simulink model "px4_controller_demo"  (R2022a)
settings: Solver=FixedStepAuto  StartTime=0.0  StopTime=inf  RelTol=1e-3  EnableMultiTasking=on
undefined symbols (not defined in the file): AUX, dev, DiscIntNeverNeededParam, dt, Main, pwm_output0, pwm_output1
libraries: simulink x8, px4lib x7, slpidlib x5, px4uORBlib x3, simulink_extras x2, sharedtransform x1, px4Sensorslib x1
settings Model: SimulationMode=external  ExtModeTrigDuration=10  Creator=The MathWorks, Inc.  LastModifiedBy=18395
settings SolverCC: AlgebraicLoopSolver=TrustRegion  PositivePriorityOrder=on  MaxZcPerStep=1
settings OptimizationCC: EnhancedBackFolding=on  PassReuseOutputArgsAs=Individual arguments  MaxStackSize=64  OptimizeBlockOrder=speed  DifferentSizesBufferReuse=on  OptimizationCustomize=off  EfficientTunableParamExpr=on
settings DebuggingCC: ParameterTunabilityLossMsg=error  UnconnectedInputMsg=warning  UnconnectedOutputMsg=warning  UnconnectedLineMsg=warning  SFMachineParentedDataDiag=warning  ArithmeticOperatorsInVariantConditions=warning
settings HardwareCC: ProdBitPerPointer=32  ProdBitPerSizeT=32  ProdBitPerPtrDiffT=32  ProdLargestAtomicInteger=Long  ProdLargestAtomicFloat=Double  ProdWordSize=32  ProdLongLongMode=on  ProdHWDeviceType=ARM Compatible->ARM Cortex
settings SFSimCC: MATLABDynamicMemAlloc=off  SimTargetLang=C++
settings RTWCC: SystemTargetFile=ert.tlc  HardwareBoard=PX4 Pixhawk 4  TLCOptions="-aInlineSetEventsForThisBaseRateFcn=TLC_FALSE -aSuppressMultiTaskScheduler=TLC_FALSE  -aRateBasedStepFcn=0"  TemplateMakefile=ert_default_tmf  GenerateReport=on  Toolchain=GNU Tools for PX4 Autopilots  IncludeHyperlinkInReport=on  LaunchReport=on  TargetLang=C++  GenerateTraceInfo=on  GenerateTraceReport=on  GenerateTraceReportSl=on  GenerateTraceReportSf=on  GenerateTraceReportEml=on  DLArmComputeVersion=19.05
settings CodeAppCC: ForceParamTrailComments=on  IgnoreCustomStorageClasses=off  OperatorAnnotations=on  SimulinkDataObjDesc=on  SFDataObjDesc=on  InsertBlockDesc=on
settings ERTTargetCC: ExtModeTransport=3  ExtModeStaticAlloc=on  ExtModeStaticAllocSize=1024  ExtModeMexFile=ext_xcp  ExtModeIntrfLevel=Level2 - Open

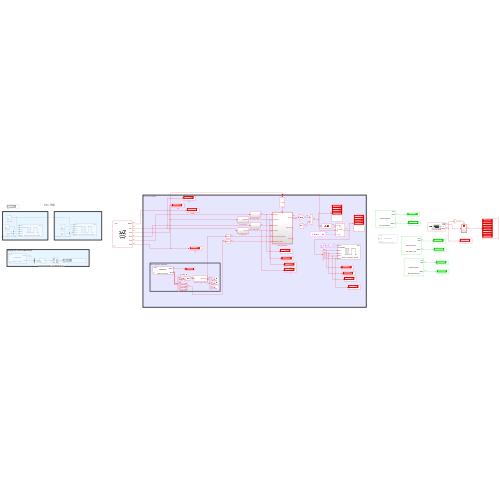
[thumbnail: Simulink's stored preview of the top-level diagram]
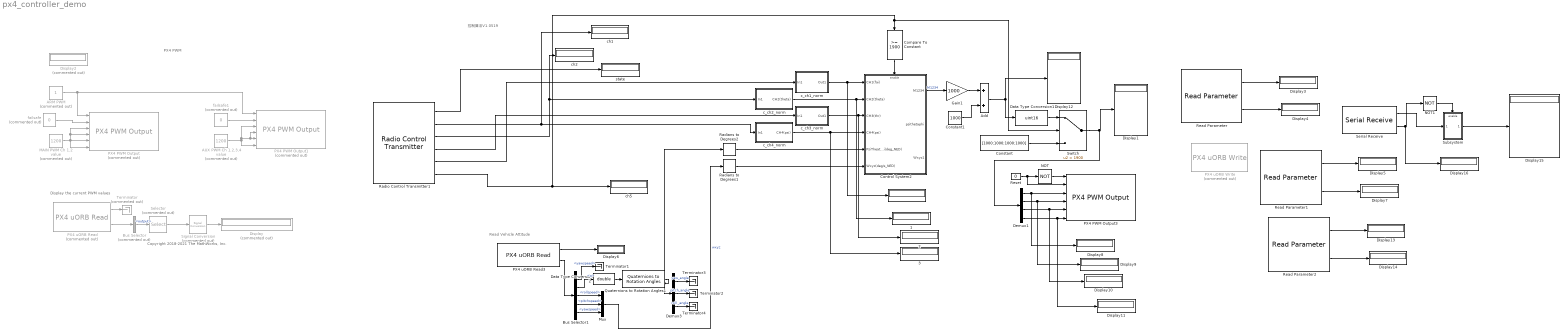
== system px4_controller_demo ==
  note: Copyright 2018-2021 The MathWorks, Inc.
  note: PX4 PWM
  note: Display the current PWM values
  note: 控制算法V1.0519
  note: Read Vehicle Attitude
    {,1..3} (4 alike) : Display
  ARM PWM : Constant  Commented=on  OutDataTypeStr=boolean  SampleTime=0.01
  AUX PWM Ch 1,2,3,4 value : Constant  Commented=on  Value=1200  OutDataTypeStr=uint16  SampleTime=0.01
  Add : Sum
  Bus Selector : BusSelector  Commented=on  OutputSignals=output
  Bus Selector1 : BusSelector  OutputSignals=yawspeed,q,rollspeed,pitchspeed,yawspeed
  Compare To Constant : simulink/Logic and Bit Operations/Compare To Constant  relop=>=  const=1900  OutDataTypeStr=boolean
  Constant : Constant  Value=[1000;1000;1000;1000]  OutDataTypeStr=uint16
  Constant1 : Constant  Value=1000  SampleTime=-1
  Control System2 : Subsystem
  Data Type Conversion1 : DataTypeConversion  OutDataTypeStr=uint16  SaturateOnIntegerOverflow=off  RndMeth=Floor
  Data Type Conversion2 : DataTypeConversion  OutDataTypeStr=double  SaturateOnIntegerOverflow=off  RndMeth=Floor
  Demux1 : Demux
  Demux3 : Demux  Outputs=3
  Display : Display  Commented=on
  Display{1,3..16} (15 alike) : Display
  Display2 : Display  Commented=on
  Gain1 : Gain  Gain=1000
  MAIN PWM Ch 1,2 value : Constant  Commented=on  Value=1200  OutDataTypeStr=uint16  SampleTime=0.01
  Mux : Mux  Inputs=3
  NOT : Logic  Operator=NOT  IconShape=distinctive  AllPortsSameDT=off  OutDataTypeStr=boolean
  NOT1 : Logic  Operator=NOT  IconShape=distinctive  AllPortsSameDT=off  OutDataTypeStr=boolean
  PX4 PWM Output : px4lib/PX4 PWM Output  Commented=on  pwmDevice=Main (/dev/pwm_output0)  pwmChannel1_=on  pwmChannel2_=on  pwmChannel3_=on  pwmChannel4_=on  pwmChannel5_=off  pwmChannel6_=off  pwmChannel7_=off  pwmChannel8_=off  forceTerminateFailsafe=off  outputErrorStatus=off
      settings: SourceProductBaseCode=PX4AUTOPILOTS
  PX4 PWM Output1 : px4lib/PX4 PWM Output  Commented=on  pwmDevice=AUX (/dev/pwm_output1)  pwmChannel1_=on  pwmChannel2_=on  pwmChannel3_=on  pwmChannel4_=on  pwmChannel5_=off  pwmChannel6_=off  pwmChannel7_=off  pwmChannel8_=off  forceTerminateFailsafe=off  outputErrorStatus=off
      settings: SourceProductBaseCode=PX4AUTOPILOTS
  PX4 PWM Output3 : px4lib/PX4 PWM Output  pwmDevice=Main (/dev/pwm_output0)  pwmChannel1_=on  pwmChannel2_=on  pwmChannel3_=on  pwmChannel4_=on  pwmChannel5_=off  pwmChannel6_=off  pwmChannel7_=off  pwmChannel8_=off  forceTerminateFailsafe=off  outputErrorStatus=off
      settings: SourceProductBaseCode=PX4AUTOPILOTS
  PX4 uORB Read : px4uORBlib/PX4 uORB Read  Commented=on  uORBTopic=actuator_outputs  selectInstance=actuator_outputs  SampleTime=0.01  BlockingMode=off  BlockTimeout=1e-3
      settings: SourceProductBaseCode=PX4AUTOPILOTS
  PX4 uORB Read3 : px4uORBlib/PX4 uORB Read  uORBTopic=vehicle_odometry  selectInstance=vehicle_odometry  SampleTime=0.01  BlockingMode=off  BlockTimeout=1e-3
      settings: SourceProductBaseCode=PX4AUTOPILOTS
  PX4 uORB Write : px4uORBlib/PX4 uORB Write  Commented=on  uORBTopic=vehicle_gps_position  selectInstance=vehicle_gps_position  MessageQueueLen=1
      settings: SourceProductBaseCode=PX4AUTOPILOTS
  Quaternions to Rotation Angles1 : sharedtransform/Quaternions to Rotation Angles  rotationOrder=ZYX  aMode=aMode
      settings: SourceProductBaseCode=AE,PW,DR,MT,VE
  Radians to Degrees1 : simulink_extras/Transformations/Radians to Degrees
  Radians to Degrees2 : simulink_extras/Transformations/Radians to Degrees
  Radio Control Transmitter1 : px4Sensorslib/Radio Control Transmitter  channel1=on  channel2=on  channel3=on  channel4=on  channel5=on  channel6=off  channel7=off  channel8=off  channel_count=off  rssi=off  rc_input_source=off  timestamp_last_signal=off  time_stamp=off  sampleTime=-1  BlockingMode=off  BlockTimeout=5
      settings: SourceProductBaseCode=PX4AUTOPILOTS
  Read Parameter : px4lib/Read Parameter  ParameterName=MC_ROLLRATE_I  DataType=FLOAT  SampleTime=0.5
      settings: SourceProductBaseCode=PX4AUTOPILOTS
  Read Parameter1 : px4lib/Read Parameter  ParameterName=FW_MAN_P_SC  DataType=FLOAT  SampleTime=0.5
      settings: SourceProductBaseCode=PX4AUTOPILOTS
  Read Parameter2 : px4lib/Read Parameter  ParameterName=MC_ROLLRATE_K  DataType=FLOAT  SampleTime=0.5
      settings: SourceProductBaseCode=PX4AUTOPILOTS
  Reset : Constant  Value=0  OutDataTypeStr=boolean
  Selector : Selector  Commented=on  InputPortWidth=16  IndexOptions=Index vector (dialog)  Indices=[1 2]  OutputSizes=1
  Serial Receive : px4lib/Serial Receive  SCIModule=/dev/ttyS2  DataType=double  DataLength=8  OutputStatus=on  SampleTime=-1  BlockingMode=off  PartialData=off  Timeout=5
      settings: SourceProductBaseCode=PX4AUTOPILOTS
  Signal Conversion : SignalConversion  Commented=on  OverrideOpt=off
  Subsystem : Subsystem
  Switch : Switch  Criteria=u2 > Threshold  Threshold=1900  SaturateOnIntegerOverflow=off  InputSameDT=off
  Terminator : Terminator  Commented=on
  Terminator{1..4} (4 alike) : Terminator
  c_ch1_norm : Subsystem
  c_ch2_norm : Subsystem
  c_ch3_norm : Subsystem
  c_ch4_norm : Subsystem
  ch1 : Display
  ch2 : Display
  ch5 : Display
  failsafe : Constant  Commented=on  Value=0  OutDataTypeStr=boolean  SampleTime=0.01
  failsafe1 : Constant  Commented=on  Value=0  OutDataTypeStr=boolean  SampleTime=0.01
  state : Display
  wires:
  failsafe/1 -> PX4 PWM Output/2
  MAIN PWM Ch 1,2 value/1 -> PX4 PWM Output/6, PX4 PWM Output/4, PX4 PWM Output/3, PX4 PWM Output/5
  PX4 uORB Read/1 -> Terminator/1
  PX4 uORB Read/2 -> Bus Selector/1
  Bus Selector/1 -> Selector/1  "<output>"
  Selector/1 -> Signal Conversion/1
  failsafe1/1 -> PX4 PWM Output1/2
  ARM PWM/1 -> PX4 PWM Output1/1, PX4 PWM Output/1
  AUX PWM Ch 1,2,3,4 value/1 -> PX4 PWM Output1/3, PX4 PWM Output1/5, PX4 PWM Output1/4, PX4 PWM Output1/6
  Signal Conversion/1 -> Display/1
  Bus Selector1/4 -> Mux/2  "<pitchspeed>"
  Radio Control Transmitter1/5 -> c_ch1_norm/1(In1)
  Gain1/1 -> Add/1
  Radio Control Transmitter1/4 -> c_ch3_norm/1(In1)
  Reset/1 -> PX4 PWM Output3/2, NOT/1
  Radio Control Transmitter1/1 -> state/1
  Demux3/2 -> Terminator2/1  "pitch_angle"
  PX4 uORB Read3/2 -> Bus Selector1/1
  Demux1/3 -> Display10/1, PX4 PWM Output3/5
  Demux1/4 -> Display11/1, PX4 PWM Output3/6
  NOT/1 -> PX4 PWM Output3/1
  Quaternions to Rotation Angles1/1 -> Demux3/1, Radians to Degrees2/1
  Data Type Conversion2/1 -> Quaternions to Rotation Angles1/1
  Demux1/1 -> Display8/1, PX4 PWM Output3/3
  Demux3/3 -> Terminator4/1  "roll _angle"
  Control System2/1(M1234) -> Gain1/1  "M1234"
  Radio Control Transmitter1/2 -> c_ch4_norm/1(In1), ch1/1
  Radians to Degrees2/1 -> Control System2/5(PsiTheatphi(deg_NED))
  Mux/1 -> Radians to Degrees1/1  "wxyz"
  PX4 uORB Read3/1 -> Display6/1
  Radians to Degrees1/1 -> Control System2/6(Wxyz(deg/s_NED))
  Data Type Conversion1/1 -> Switch/1
  Bus Selector1/3 -> Mux/1  "<rollspeed>"
  Add/1 -> Data Type Conversion1/1, Display12/1
  Bus Selector1/2 -> Data Type Conversion2/1  "<q>"
  Constant1/1 -> Add/2
  Demux3/1 -> Terminator3/1  "yaw_angle"
  Radio Control Transmitter1/3 -> c_ch2_norm/1(In1), ch2/1
  Bus Selector1/5 -> Mux/3  "<yawspeed>"
  Bus Selector1/1 -> Terminator1/1  "<yawspeed>"
  c_ch3_norm/1(Out1) -> "  2"/1, Control System2/3(CH3(thr))
  c_ch2_norm/1(CH2(theta)) -> "  1"/1, Control System2/2(CH2(theta))
  c_ch4_norm/1(CH4(psi)) -> "  3"/1, Control System2/4(CH4(psi))
  c_ch1_norm/1(Out1) -> "  "/1, Control System2/1(CH1(fai))
  Demux1/2 -> Display9/1, PX4 PWM Output3/4
  Radio Control Transmitter1/6 -> ch5/1, Compare To Constant/1, Switch/2
  Compare To Constant/1 -> Control System2/Enable
  Switch/1 -> Demux1/1, Display1/1
  Constant/1 -> Switch/3
  Read Parameter/1 -> Display3/1
  Read Parameter/2 -> Display4/1
  Read Parameter1/2 -> Display7/1
  Read Parameter1/1 -> Display5/1
  Read Parameter2/1 -> Display13/1
  Read Parameter2/2 -> Display14/1
  Serial Receive/2 -> Display16/1, NOT1/1
  Serial Receive/1 -> Subsystem/1(In1)
  Subsystem/1(Out1) -> Display15/1
  NOT1/1 -> Subsystem/Enable

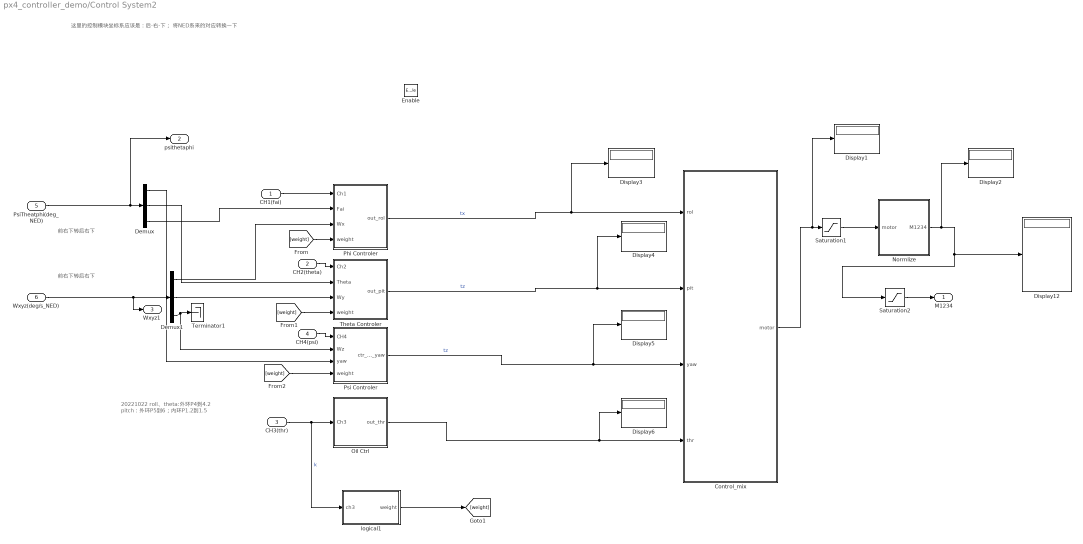
== system px4_controller_demo/Control System2 ==
  note: 20221022
      | roll、theta:外环P4到4.2
      | pitch：外环P5到6；内环P1.2到1.5
  note: 前右下转后右下
  note: 这里的控制模块坐标系应该是：后-右-下；
      | 将NED系来的对应转换一下
  note: 前右下转后右下
  CH1(fai) : Inport
  CH2(theta) : Inport  Port=2
  CH3(thr) : Inport  Port=3
  CH4(psi) : Inport  Port=4
  PsiTheatphi(deg_NED) : Inport  Port=5
  Wxyz(deg/s_NED) : Inport  Port=6
  Enable : EnablePort
  Control_mix : MATLAB Function  TreatAsAtomicUnit=on
  Demux : Demux  Outputs=3
  Demux1 : Demux  Outputs=3
  Display{1..6,12} (7 alike) : Display
  Normlize : Subsystem
  Oil Ctrl : Subsystem
  Phi Controler : Subsystem
  Psi Controler : Subsystem
  Saturation1 : Saturate  UpperLimit=1000  LowerLimit=0
  Saturation2 : Saturate  UpperLimit=1  LowerLimit=0
  Terminator1 : Terminator
  Theta Controler : Subsystem
  logical1 : Subsystem
  M1234 : Outport
  psithetaphi : Outport  Port=2
  Wxyz1 : Outport  Port=3
  wires:
  Demux1/3 -> Psi Controler/2(Wz), Terminator1/1
  Wxyz(deg/s_NED)/1 -> Wxyz1/1, Demux1/1
  PsiTheatphi(deg_NED)/1 -> psithetaphi/1, Demux/1
  CH2(theta)/1 -> Theta Controler/1(Ch2)
  CH4(psi)/1 -> Psi Controler/1(CH4)
  CH1(fai)/1 -> Phi Controler/1(Ch1)
  Demux1/1 -> Phi Controler/3(Wx)
  Demux1/2 -> Theta Controler/3(Wy)
  Demux/3 -> Phi Controler/2(Fai)
  Demux/2 -> Theta Controler/2(Theta)
  Saturation1/1 -> Normlize/1(motor)
  Normlize/1(M1234) -> Display2/1, Display12/1, Saturation2/1
  Saturation2/1 -> M1234/1
  Control_mix/1(motor) -> Display1/1, Saturation1/1
  Psi Controler/1(ctr_out_yaw) -> Display5/1, Control_mix/3(yaw)  "tz"
  Phi Controler/1(out_rol) -> Display3/1, Control_mix/1(rol)  "tx"
  Theta Controler/1(out_pit) -> Display4/1, Control_mix/2(pit)  "tz"
  Demux/1 -> Psi Controler/3(yaw)
  CH3(thr)/1 -> logical1/1(ch3), Oil Ctrl/1(Ch3)  "k"
  logical1/1(weight) -> [weight]
  [weight] -> Phi Controler/4(weight)
  [weight] -> Theta Controler/4(weight)
  [weight] -> Psi Controler/4(weight)
  Oil Ctrl/1(out_thr) -> Display6/1, Control_mix/4(thr)

== system px4_controller_demo/Subsystem ==
  In1 : Inport
  Enable : EnablePort
  Out1 : Outport
  wires:
  In1/1 -> Out1/1

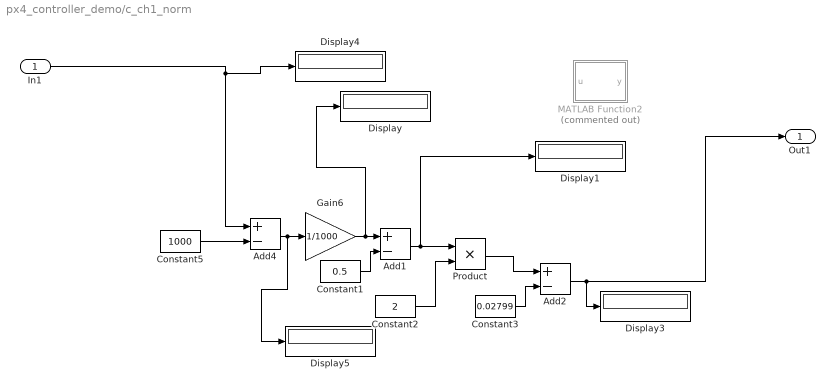
== system px4_controller_demo/c_ch1_norm ==
  In1 : Inport
  Add1 : Sum  Inputs=+-
  Add2 : Sum  Inputs=+-
  Add4 : Sum  Inputs=+-  AccumDataTypeStr=uint16
  Constant1 : Constant  Value=0.5
  Constant2 : Constant  Value=2  OutDataTypeStr=uint16
  Constant3 : Constant  Value=0.02799  OutDataTypeStr=uint16
  Constant5 : Constant  Value=1000  OutDataTypeStr=uint16
  Display{,1,3..5} (5 alike) : Display
  Gain6 : Gain  Gain=1/1000
  MATLAB Function2 : MATLAB Function  Commented=on  TreatAsAtomicUnit=on
  Product : Product
  Out1 : Outport
  wires:
  Add4/1 -> Display5/1, Gain6/1
  Constant5/1 -> Add4/2
  Gain6/1 -> Display/1, Add1/1
  In1/1 -> Display4/1, Add4/1
  Constant1/1 -> Add1/2
  Add1/1 -> Display1/1, Product/1
  Constant2/1 -> Product/2
  Product/1 -> Add2/1
  Constant3/1 -> Add2/2
  Add2/1 -> Display3/1, Out1/1

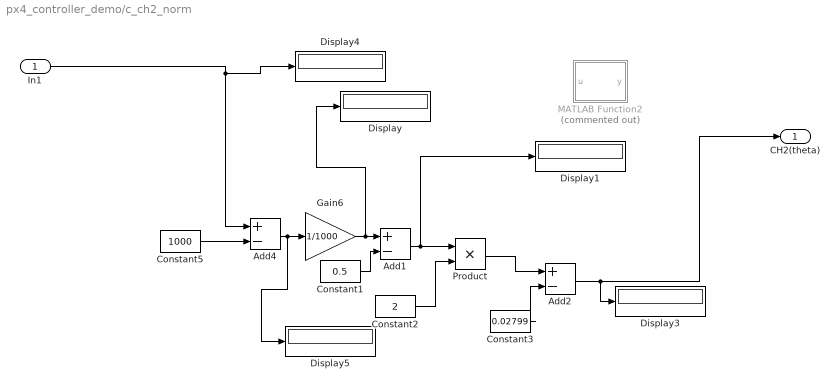
== system px4_controller_demo/c_ch2_norm ==
  In1 : Inport
  Add1 : Sum  Inputs=+-
  Add2 : Sum  Inputs=+-
  Add4 : Sum  Inputs=+-  AccumDataTypeStr=uint16
  Constant1 : Constant  Value=0.5
  Constant2 : Constant  Value=2  OutDataTypeStr=uint16
  Constant3 : Constant  Value=0.02799  OutDataTypeStr=uint16
  Constant5 : Constant  Value=1000  OutDataTypeStr=uint16
  Display{,1,3..5} (5 alike) : Display
  Gain6 : Gain  Gain=1/1000
  MATLAB Function2 : MATLAB Function  Commented=on  TreatAsAtomicUnit=on
  Product : Product
  CH2(theta) : Outport
  wires:
  Constant1/1 -> Add1/2
  Add1/1 -> Display1/1, Product/1
  Gain6/1 -> Display/1, Add1/1
  In1/1 -> Display4/1, Add4/1
  Add4/1 -> Display5/1, Gain6/1
  Constant2/1 -> Product/2
  Constant5/1 -> Add4/2
  Constant3/1 -> Add2/2
  Product/1 -> Add2/1
  Add2/1 -> Display3/1, CH2(theta)/1

== system px4_controller_demo/c_ch3_norm ==
  In1 : Inport
  Add2 : Sum  Inputs=+-
  Add4 : Sum  Inputs=+-  AccumDataTypeStr=uint16
  Constant3 : Constant  Value=0.095  OutDataTypeStr=uint16
  Constant5 : Constant  Value=1000  OutDataTypeStr=uint16
  Display : Display
  Display4 : Display
  Gain6 : Gain  Gain=1/1000
  Out1 : Outport
  wires:
  In1/1 -> Display4/1, Add4/1
  Add4/1 -> Gain6/1
  Constant5/1 -> Add4/2
  Constant3/1 -> Add2/2
  Gain6/1 -> Add2/1
  Add2/1 -> Display/1, Out1/1

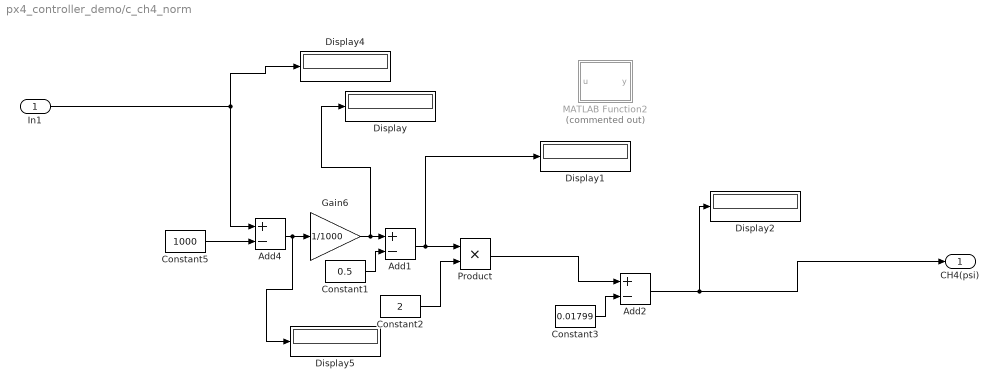
== system px4_controller_demo/c_ch4_norm ==
  In1 : Inport
  Add1 : Sum  Inputs=+-
  Add2 : Sum  Inputs=+-
  Add4 : Sum  Inputs=+-  AccumDataTypeStr=uint16
  Constant1 : Constant  Value=0.5
  Constant2 : Constant  Value=2  OutDataTypeStr=uint16
  Constant3 : Constant  Value=0.01799  OutDataTypeStr=uint16
  Constant5 : Constant  Value=1000  OutDataTypeStr=uint16
  Display{,1..2,4..5} (5 alike) : Display
  Gain6 : Gain  Gain=1/1000
  MATLAB Function2 : MATLAB Function  Commented=on  TreatAsAtomicUnit=on
  Product : Product
  CH4(psi) : Outport
  wires:
  Constant1/1 -> Add1/2
  Add1/1 -> Display1/1, Product/1
  Gain6/1 -> Display/1, Add1/1
  In1/1 -> Display4/1, Add4/1
  Add4/1 -> Display5/1, Gain6/1
  Constant2/1 -> Product/2
  Constant5/1 -> Add4/2
  Constant3/1 -> Add2/2
  Product/1 -> Add2/1
  Add2/1 -> Display2/1, CH4(psi)/1

== system px4_controller_demo/Control System2/Normlize ==
  motor : Inport
  Constant : Constant  Value=1000
  Divide : Product  Inputs=*/
  M1234 : Outport
  wires:
  Constant/1 -> Divide/2
  motor/1 -> Divide/1
  Divide/1 -> M1234/1

== system px4_controller_demo/Control System2/Oil Ctrl ==
  note: ch3油门归一化为[0 1,若ch3开度高于0.4，油门量足够俯仰滚转才能驱的动]
  Ch3 : Inport
  Gain : Gain  Gain=1000
  Max ExpRate1 : Saturate  UpperLimit=1000  LowerLimit=0
  out_thr : Outport
  wires:
  Ch3/1 -> Gain/1  "k"
  Max ExpRate1/1 -> out_thr/1
  Gain/1 -> Max ExpRate1/1

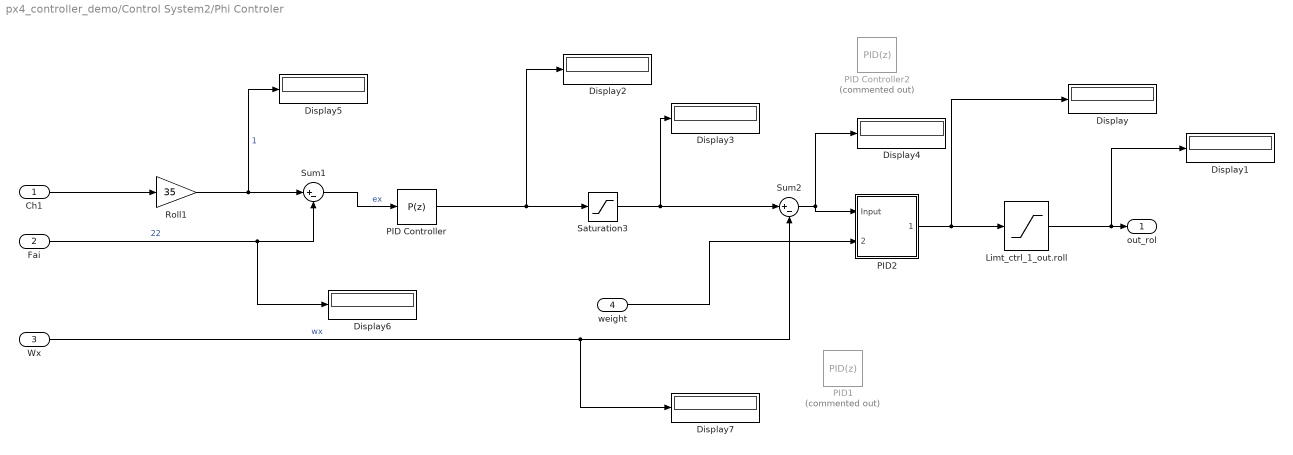
== system px4_controller_demo/Control System2/Phi Controler ==
  Ch1 : Inport
  Fai : Inport  Port=2
  Wx : Inport  Port=3
  weight : Inport  Port=4
  Display{,1..7} (8 alike) : Display
  Limt_ctrl_1_out.roll : Saturate  UpperLimit=1000  LowerLimit=-1000
  PID Controller : slpidlib/PID Controller  Controller=P  Form=Parallel  TimeDomain=Discrete-time  UseExternalTs=off  SampleTime=-1  IntegratorMethod=Forward Euler  FilterMethod=Forward Euler  ControllerParametersSource=internal  P=4  I=1  UseKiTs=off  D=0  N=100  UseFilter=on  TunerSelectOption=Transfer Function Based (PID Tuner App)  InitialConditionSource=internal  InitialConditionForIntegrator=0  InitialConditionForFilter=0  DifferentiatorICPrevScaledInput=0  ExternalReset=none  TrackingMode=off  Kt=1  LimitOutput=off  SatLimitsSource=internal  UpperSaturationLimit=inf  LowerSaturationLimit=-inf  LinearizeAsGain=on  AntiWindupMode=none  Kb=1  POutMin=[]  POutMax=[]  IOutMin=[]  IOutMax=[]  DOutMin=[]  DOutMax=[]  NOutMin=[]  NOutMax=[]  SumOutMin=[]  SumOutMax=[]  SaturationOutMin=[]  SaturationOutMax=[]  PParamMin=[]  PParamMax=[]  IParamMin=[]  IParamMax=[]  DParamMin=[]  DParamMax=[]  NParamMin=[]  NParamMax=[]  KbParamMin=[]  KbParamMax=[]  KtParamMin=[]  KtParamMax=[]  KbOutMin=[]  KbOutMax=[]  KtOutMin=[]  KtOutMax=[]  IntegratorOutMin=[]  IntegratorOutMax=[]  FilterOutMin=[]  FilterOutMax=[]  SumI1OutMin=[]  SumI1OutMax=[]  SumI2OutMin=[]  SumI2OutMax=[]  SumI3OutMin=[]  SumI3OutMax=[]  SumI4OutMin=[]  SumI4OutMax=[]  SumDOutMin=[]  SumDOutMax=[]  DifferentiatorOutMin=[]  DifferentiatorOutMax=[]  FilterDiffOutCoefMin=[]  FilterDiffOutCoefMax=[]  ReciprocalOutMin=[]  ReciprocalOutMax=[]  SumDenOutMin=[]  SumDenOutMax=[]  SumNumOutMin=[]  SumNumOutMax=[]  DivideOutMin=[]  DivideOutMax=[]  UdiffTsProdOutMin=[]  UdiffTsProdOutMax=[]  NTsProdOutMin=[]  NTsProdOutMax=[]  UintegralTsProdOutMin=[]  UintegralTsProdOutMax=[]  UngainTsProdOutMin=[]  UngainTsProdOutMax=[]  IntegratorContinuousStateAttributes=''  IntegratorStateMustResolveToSignalObject=off  IntegratorRTWStateStorageClass=Auto  FilterContinuousStateAttributes=''  FilterStateMustResolveToSignalObject=off  FilterRTWStateStorageClass=Auto  ParallelPVariant=InternalParameters  IdealPVariant=Disabled  IVariant=Disabled  DVariant=Disabled  IntegratorVariant=Disabled  SatVariant=Disabled  AWVariant=Disabled  PCopyVariant=Disabled  TRVariant=Disabled  FdbkBlocksVariant=Forward  IdealPFdbkVariant=Disabled  SatFdbkVariant=Disabled  DerivativeFilterVariant=Disabled  NVariant=Disabled  NCopyVariant=Disabled_SignalSpec  FilterICVariant=Disabled  IntegratorICVariant=Disabled  ExternalResetVariant=Disabled  TRSumVariant=Passthrough  SumFdbkVariant=Disabled  SumVariant=Passthrough_P  TsampFilterVariant=InternalTs  TsampNgainVariant=Passthrough  TsampIntegralVariant=Disabled_SignalSpec  ExternalSaturationOutDataTypeStr=Inherit: Same as second input  aMode=0
  PID Controller2 : slpidlib/PID Controller  Commented=on  Controller=PID  Form=Parallel  TimeDomain=Discrete-time  UseExternalTs=off  SampleTime=-1  IntegratorMethod=Forward Euler  FilterMethod=Forward Euler  ControllerParametersSource=internal  P=0.8  I=1.2  UseKiTs=off  D=0.03  N=100  UseFilter=on  TunerSelectOption=Transfer Function Based (PID Tuner App)  InitialConditionSource=internal  InitialConditionForIntegrator=0  InitialConditionForFilter=0  DifferentiatorICPrevScaledInput=0  ExternalReset=none  TrackingMode=off  Kt=1  LimitOutput=off  SatLimitsSource=internal  UpperSaturationLimit=inf  LowerSaturationLimit=-inf  LinearizeAsGain=on  AntiWindupMode=none  Kb=1  POutMin=[]  POutMax=[]  IOutMin=[]  IOutMax=[]  DOutMin=[]  DOutMax=[]  NOutMin=[]  NOutMax=[]  SumOutMin=[]  SumOutMax=[]  SaturationOutMin=[]  SaturationOutMax=[]  PParamMin=[]  PParamMax=[]  IParamMin=[]  IParamMax=[]  DParamMin=[]  DParamMax=[]  NParamMin=[]  NParamMax=[]  KbParamMin=[]  KbParamMax=[]  KtParamMin=[]  KtParamMax=[]  KbOutMin=[]  KbOutMax=[]  KtOutMin=[]  KtOutMax=[]  IntegratorOutMin=[]  IntegratorOutMax=[]  FilterOutMin=[]  FilterOutMax=[]  SumI1OutMin=[]  SumI1OutMax=[]  SumI2OutMin=[]  SumI2OutMax=[]  SumI3OutMin=[]  SumI3OutMax=[]  SumI4OutMin=[]  SumI4OutMax=[]  SumDOutMin=[]  SumDOutMax=[]  DifferentiatorOutMin=[]  DifferentiatorOutMax=[]  FilterDiffOutCoefMin=[]  FilterDiffOutCoefMax=[]  ReciprocalOutMin=[]  ReciprocalOutMax=[]  SumDenOutMin=[]  SumDenOutMax=[]  SumNumOutMin=[]  SumNumOutMax=[]  DivideOutMin=[]  DivideOutMax=[]  UdiffTsProdOutMin=[]  UdiffTsProdOutMax=[]  NTsProdOutMin=[]  NTsProdOutMax=[]  UintegralTsProdOutMin=[]  UintegralTsProdOutMax=[]  UngainTsProdOutMin=[]  UngainTsProdOutMax=[]  IntegratorContinuousStateAttributes=''  IntegratorStateMustResolveToSignalObject=off  IntegratorRTWStateStorageClass=Auto  FilterContinuousStateAttributes=''  FilterStateMustResolveToSignalObject=off  FilterRTWStateStorageClass=Auto  ParallelPVariant=InternalParameters  IdealPVariant=Disabled  IVariant=InternalParameters  DVariant=InternalParameters  IntegratorVariant=Discrete  SatVariant=Disabled  AWVariant=Passthrough  PCopyVariant=Disabled  TRVariant=Disabled  FdbkBlocksVariant=Forward  IdealPFdbkVariant=Disabled  SatFdbkVariant=Disabled  DerivativeFilterVariant=ForwardEulerFilter  NVariant=InternalParameters  NCopyVariant=Disabled  FilterICVariant=InternalICsFilter  IntegratorICVariant=InternalICs  ExternalResetVariant=Disabled  TRSumVariant=Passthrough  SumFdbkVariant=Disabled  SumVariant=Sum_PID  TsampFilterVariant=InternalTs  TsampNgainVariant=Passthrough  TsampIntegralVariant=Passthrough  ExternalSaturationOutDataTypeStr=Inherit: Same as second input  aMode=0
  PID1 : slpidlib/PID Controller  Commented=on  Controller=PID  Form=Parallel  TimeDomain=Discrete-time  UseExternalTs=off  SampleTime=-1  IntegratorMethod=Backward Euler  FilterMethod=Forward Euler  ControllerParametersSource=internal  P=0.8  I=1.2  UseKiTs=off  D=0.03  N=50  UseFilter=on  TunerSelectOption=Transfer Function Based (PID Tuner App)  InitialConditionSource=internal  InitialConditionForIntegrator=0  InitialConditionForFilter=0  DifferentiatorICPrevScaledInput=0  ExternalReset=none  TrackingMode=off  Kt=1  LimitOutput=on  SatLimitsSource=internal  UpperSaturationLimit=1000  LowerSaturationLimit=-1000  LinearizeAsGain=off  AntiWindupMode=none  Kb=1  POutMin=[]  POutMax=[]  IOutMin=[]  IOutMax=[]  DOutMin=[]  DOutMax=[]  NOutMin=[]  NOutMax=[]  SumOutMin=[]  SumOutMax=[]  SaturationOutMin=[]  SaturationOutMax=[]  PParamMin=[]  PParamMax=[]  IParamMin=[]  IParamMax=[]  DParamMin=[]  DParamMax=[]  NParamMin=[]  NParamMax=[]  KbParamMin=[]  KbParamMax=[]  KtParamMin=[]  KtParamMax=[]  KbOutMin=[]  KbOutMax=[]  KtOutMin=[]  KtOutMax=[]  IntegratorOutMin=[]  IntegratorOutMax=[]  FilterOutMin=[]  FilterOutMax=[]  SumI1OutMin=[]  SumI1OutMax=[]  SumI2OutMin=[]  SumI2OutMax=[]  SumI3OutMin=[]  SumI3OutMax=[]  SumI4OutMin=[]  SumI4OutMax=[]  SumDOutMin=[]  SumDOutMax=[]  DifferentiatorOutMin=[]  DifferentiatorOutMax=[]  FilterDiffOutCoefMin=[]  FilterDiffOutCoefMax=[]  ReciprocalOutMin=[]  ReciprocalOutMax=[]  SumDenOutMin=[]  SumDenOutMax=[]  SumNumOutMin=[]  SumNumOutMax=[]  DivideOutMin=[]  DivideOutMax=[]  UdiffTsProdOutMin=[]  UdiffTsProdOutMax=[]  NTsProdOutMin=[]  NTsProdOutMax=[]  UintegralTsProdOutMin=[]  UintegralTsProdOutMax=[]  UngainTsProdOutMin=[]  UngainTsProdOutMax=[]  IntegratorContinuousStateAttributes=''  IntegratorStateMustResolveToSignalObject=off  IntegratorRTWStateStorageClass=Auto  FilterContinuousStateAttributes=''  FilterStateMustResolveToSignalObject=off  FilterRTWStateStorageClass=Auto  ParallelPVariant=InternalParameters  IdealPVariant=Disabled  IVariant=InternalParameters  DVariant=InternalParameters  IntegratorVariant=Discrete  SatVariant=Enabled  AWVariant=Passthrough  PCopyVariant=Disabled  TRVariant=Disabled  FdbkBlocksVariant=Forward  IdealPFdbkVariant=Disabled  SatFdbkVariant=Disabled  DerivativeFilterVariant=ForwardEulerFilter  NVariant=InternalParameters  NCopyVariant=Disabled  FilterICVariant=InternalICsFilter  IntegratorICVariant=InternalICs  ExternalResetVariant=Disabled  TRSumVariant=Passthrough  SumFdbkVariant=Disabled  SumVariant=Sum_PID  TsampFilterVariant=InternalTs  TsampNgainVariant=Passthrough  TsampIntegralVariant=Passthrough  ExternalSaturationOutDataTypeStr=Inherit: Same as second input  aMode=0
  PID2 : Subsystem
  Roll1 : Gain  Gain=35
  Saturation3 : Saturate  UpperLimit=300  LowerLimit=-300
  Sum1 : Sum  Inputs=|+-
  Sum2 : Sum  Inputs=|+-
  out_rol : Outport
  wires:
  Limt_ctrl_1_out.roll/1 -> Display1/1, out_rol/1
  Saturation3/1 -> Display3/1, Sum2/1
  PID Controller/1 -> Display2/1, Saturation3/1
  Roll1/1 -> Display5/1, Sum1/1  "1"
  Wx/1 -> Display7/1, Sum2/2  "wx"
  Fai/1 -> Display6/1, Sum1/2  "22"
  Ch1/1 -> Roll1/1
  Sum2/1 -> PID2/1(Input), Display4/1
  Sum1/1 -> PID Controller/1  "ex"
  PID2/1(Output) -> Display/1, Limt_ctrl_1_out.roll/1
  weight/1 -> PID2/2(weight)

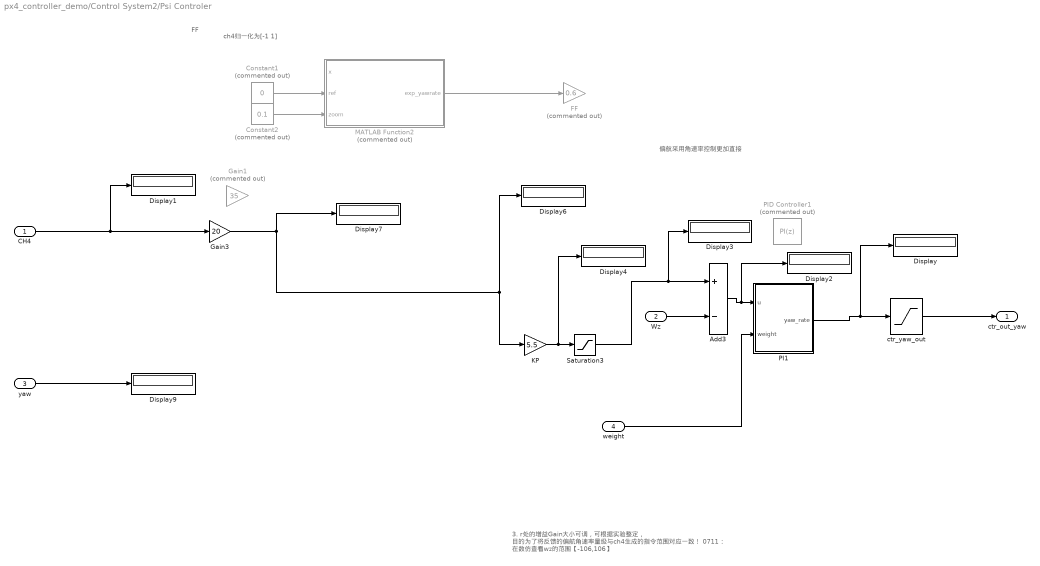
== system px4_controller_demo/Control System2/Psi Controler ==
  note: 偏航采用角速率控制更加直接
  note: 3. r处的增益Gain大小可调，可根据实验整定，
      | 目的为了将反馈的偏航角速率量级与ch4生成的指令范围对应一致！
      |
      | 0711：
      | 在数仿查看wz的范围【-106,106】
  note: FF
  note: ch4归一化为[-1 1]
  CH4 : Inport
  Wz : Inport  Port=2
  yaw : Inport  Port=3
  weight : Inport  Port=4
  Add3 : Sum  Inputs=+-
  Constant1 : Constant  Commented=on  Value=0
  Constant2 : Constant  Commented=on  Value=0.1
  Display{,1..4,6..7,9} (8 alike) : Display
  FF : Gain  Commented=on  Gain=0.6
  Gain1 : Gain  Commented=on  Gain=35
  Gain3 : Gain  Gain=20
  KP : Gain  Gain=5.5
  MATLAB Function2 : MATLAB Function  Commented=on  TreatAsAtomicUnit=on
  PI1 : Subsystem
  PID Controller1 : slpidlib/PID Controller  Commented=on  Controller=PI  Form=Parallel  TimeDomain=Discrete-time  UseExternalTs=off  SampleTime=-1  IntegratorMethod=Forward Euler  FilterMethod=Forward Euler  ControllerParametersSource=internal  P=1.4  I=0.7  UseKiTs=off  D=0  N=100  UseFilter=on  TunerSelectOption=Transfer Function Based (PID Tuner App)  InitialConditionSource=internal  InitialConditionForIntegrator=0  InitialConditionForFilter=0  DifferentiatorICPrevScaledInput=0  ExternalReset=none  TrackingMode=off  Kt=1  LimitOutput=off  SatLimitsSource=internal  UpperSaturationLimit=inf  LowerSaturationLimit=-inf  LinearizeAsGain=on  AntiWindupMode=none  Kb=1  POutMin=[]  POutMax=[]  IOutMin=[]  IOutMax=[]  DOutMin=[]  DOutMax=[]  NOutMin=[]  NOutMax=[]  SumOutMin=[]  SumOutMax=[]  SaturationOutMin=[]  SaturationOutMax=[]  PParamMin=[]  PParamMax=[]  IParamMin=[]  IParamMax=[]  DParamMin=[]  DParamMax=[]  NParamMin=[]  NParamMax=[]  KbParamMin=[]  KbParamMax=[]  KtParamMin=[]  KtParamMax=[]  KbOutMin=[]  KbOutMax=[]  KtOutMin=[]  KtOutMax=[]  IntegratorOutMin=[]  IntegratorOutMax=[]  FilterOutMin=[]  FilterOutMax=[]  SumI1OutMin=[]  SumI1OutMax=[]  SumI2OutMin=[]  SumI2OutMax=[]  SumI3OutMin=[]  SumI3OutMax=[]  SumI4OutMin=[]  SumI4OutMax=[]  SumDOutMin=[]  SumDOutMax=[]  DifferentiatorOutMin=[]  DifferentiatorOutMax=[]  FilterDiffOutCoefMin=[]  FilterDiffOutCoefMax=[]  ReciprocalOutMin=[]  ReciprocalOutMax=[]  SumDenOutMin=[]  SumDenOutMax=[]  SumNumOutMin=[]  SumNumOutMax=[]  DivideOutMin=[]  DivideOutMax=[]  UdiffTsProdOutMin=[]  UdiffTsProdOutMax=[]  NTsProdOutMin=[]  NTsProdOutMax=[]  UintegralTsProdOutMin=[]  UintegralTsProdOutMax=[]  UngainTsProdOutMin=[]  UngainTsProdOutMax=[]  IntegratorContinuousStateAttributes=''  IntegratorStateMustResolveToSignalObject=off  IntegratorRTWStateStorageClass=Auto  FilterContinuousStateAttributes=''  FilterStateMustResolveToSignalObject=off  FilterRTWStateStorageClass=Auto  ParallelPVariant=InternalParameters  IdealPVariant=Disabled  IVariant=InternalParameters  DVariant=Disabled  IntegratorVariant=Discrete  SatVariant=Disabled  AWVariant=Passthrough  PCopyVariant=Disabled  TRVariant=Disabled  FdbkBlocksVariant=Forward  IdealPFdbkVariant=Disabled  SatFdbkVariant=Disabled  DerivativeFilterVariant=Disabled  NVariant=Disabled  NCopyVariant=Disabled_SignalSpec  FilterICVariant=Disabled  IntegratorICVariant=InternalICs  ExternalResetVariant=Disabled  TRSumVariant=Passthrough  SumFdbkVariant=Disabled  SumVariant=Sum_PI  TsampFilterVariant=InternalTs  TsampNgainVariant=Passthrough  TsampIntegralVariant=Passthrough  ExternalSaturationOutDataTypeStr=Inherit: Same as second input  aMode=0
  Saturation3 : Saturate  UpperLimit=200  LowerLimit=-200
  ctr_yaw_out : Saturate  UpperLimit=800  LowerLimit=-800
  ctr_out_yaw : Outport
  wires:
  Constant1/1 -> MATLAB Function2/2(ref)
  Constant2/1 -> MATLAB Function2/3(zoom)
  ctr_yaw_out/1 -> ctr_out_yaw/1
  MATLAB Function2/1(exp_yawrate) -> FF/1
  PI1/1(yaw_rate) -> Display/1, ctr_yaw_out/1
  Add3/1 -> Display2/1, PI1/1(u)
  Wz/1 -> Add3/2
  KP/1 -> Display4/1, Saturation3/1
  Saturation3/1 -> Display3/1, Add3/1
  Gain3/1 -> Display6/1, KP/1, Display7/1
  CH4/1 -> Display1/1, Gain3/1
  yaw/1 -> Display9/1
  weight/1 -> PI1/2(weight)

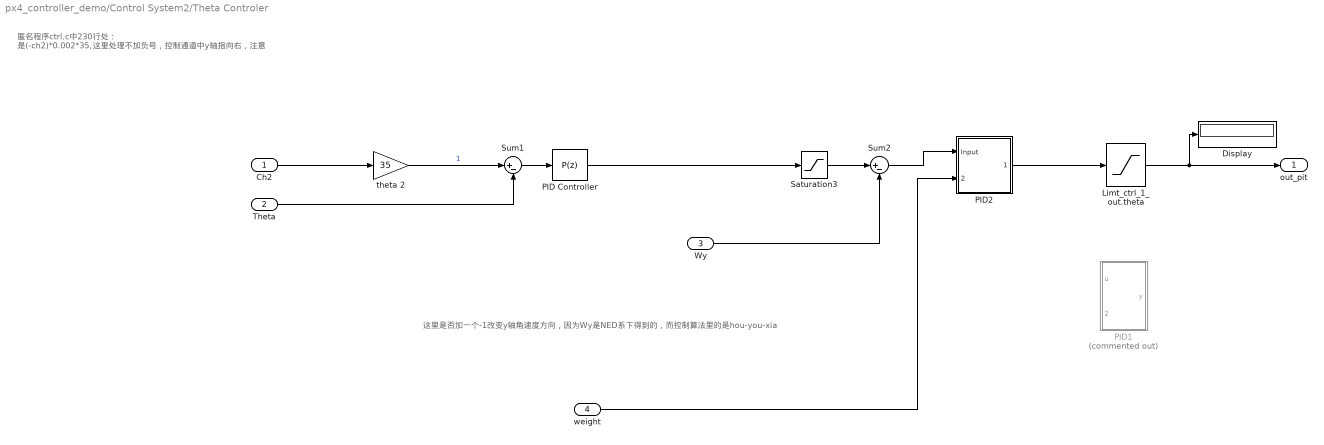
== system px4_controller_demo/Control System2/Theta Controler ==
  note: 匿名程序ctrl.c中230行处：
      | 是(-ch2)*0.002*35,这里处理不加负号，控制通道中y轴指向右，注意
  note: 这里是否加一个-1改变y轴角速度方向，因为Wy是NED系下得到的，而控制算法里的是hou-you-xia
  Ch2 : Inport
  Theta : Inport  Port=2
  Wy : Inport  Port=3
  weight : Inport  Port=4
  Display : Display
  Limt_ctrl_1_out.theta : Saturate  UpperLimit=1000  LowerLimit=-1000
  PID Controller : slpidlib/PID Controller  Controller=P  Form=Parallel  TimeDomain=Discrete-time  UseExternalTs=off  SampleTime=-1  IntegratorMethod=Forward Euler  FilterMethod=Forward Euler  ControllerParametersSource=internal  P=4  I=1  UseKiTs=off  D=0  N=100  UseFilter=on  TunerSelectOption=Transfer Function Based (PID Tuner App)  InitialConditionSource=internal  InitialConditionForIntegrator=0  InitialConditionForFilter=0  DifferentiatorICPrevScaledInput=0  ExternalReset=none  TrackingMode=off  Kt=1  LimitOutput=off  SatLimitsSource=internal  UpperSaturationLimit=inf  LowerSaturationLimit=-inf  LinearizeAsGain=on  AntiWindupMode=none  Kb=1  POutMin=[]  POutMax=[]  IOutMin=[]  IOutMax=[]  DOutMin=[]  DOutMax=[]  NOutMin=[]  NOutMax=[]  SumOutMin=[]  SumOutMax=[]  SaturationOutMin=[]  SaturationOutMax=[]  PParamMin=[]  PParamMax=[]  IParamMin=[]  IParamMax=[]  DParamMin=[]  DParamMax=[]  NParamMin=[]  NParamMax=[]  KbParamMin=[]  KbParamMax=[]  KtParamMin=[]  KtParamMax=[]  KbOutMin=[]  KbOutMax=[]  KtOutMin=[]  KtOutMax=[]  IntegratorOutMin=[]  IntegratorOutMax=[]  FilterOutMin=[]  FilterOutMax=[]  SumI1OutMin=[]  SumI1OutMax=[]  SumI2OutMin=[]  SumI2OutMax=[]  SumI3OutMin=[]  SumI3OutMax=[]  SumI4OutMin=[]  SumI4OutMax=[]  SumDOutMin=[]  SumDOutMax=[]  DifferentiatorOutMin=[]  DifferentiatorOutMax=[]  FilterDiffOutCoefMin=[]  FilterDiffOutCoefMax=[]  ReciprocalOutMin=[]  ReciprocalOutMax=[]  SumDenOutMin=[]  SumDenOutMax=[]  SumNumOutMin=[]  SumNumOutMax=[]  DivideOutMin=[]  DivideOutMax=[]  UdiffTsProdOutMin=[]  UdiffTsProdOutMax=[]  NTsProdOutMin=[]  NTsProdOutMax=[]  UintegralTsProdOutMin=[]  UintegralTsProdOutMax=[]  UngainTsProdOutMin=[]  UngainTsProdOutMax=[]  IntegratorContinuousStateAttributes=''  IntegratorStateMustResolveToSignalObject=off  IntegratorRTWStateStorageClass=Auto  FilterContinuousStateAttributes=''  FilterStateMustResolveToSignalObject=off  FilterRTWStateStorageClass=Auto  ParallelPVariant=InternalParameters  IdealPVariant=Disabled  IVariant=Disabled  DVariant=Disabled  IntegratorVariant=Disabled  SatVariant=Disabled  AWVariant=Disabled  PCopyVariant=Disabled  TRVariant=Disabled  FdbkBlocksVariant=Forward  IdealPFdbkVariant=Disabled  SatFdbkVariant=Disabled  DerivativeFilterVariant=Disabled  NVariant=Disabled  NCopyVariant=Disabled_SignalSpec  FilterICVariant=Disabled  IntegratorICVariant=Disabled  ExternalResetVariant=Disabled  TRSumVariant=Passthrough  SumFdbkVariant=Disabled  SumVariant=Passthrough_P  TsampFilterVariant=InternalTs  TsampNgainVariant=Passthrough  TsampIntegralVariant=Disabled_SignalSpec  ExternalSaturationOutDataTypeStr=Inherit: Same as second input  aMode=0
  PID1 : Subsystem  Commented=on
  PID2 : Subsystem
  Saturation3 : Saturate  UpperLimit=300  LowerLimit=-300
  Sum1 : Sum  Inputs=|+-
  Sum2 : Sum  Inputs=|+-
  theta 2 : Gain  Gain=35
  out_pit : Outport
  wires:
  Saturation3/1 -> Sum2/1
  PID Controller/1 -> Saturation3/1
  theta 2/1 -> Sum1/1  "1"
  Theta/1 -> Sum1/2
  Sum1/1 -> PID Controller/1
  Ch2/1 -> theta 2/1
  Sum2/1 -> PID2/1(Input)
  Limt_ctrl_1_out.theta/1 -> Display/1, out_pit/1
  PID2/1(Output) -> Limt_ctrl_1_out.theta/1
  Wy/1 -> Sum2/2
  weight/1 -> PID2/2(weight)

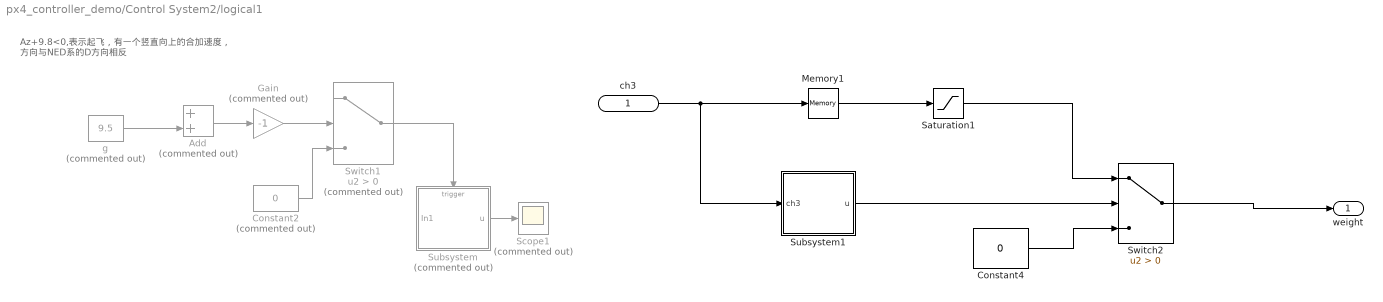
== system px4_controller_demo/Control System2/logical1 ==
  note: Az+9.8<0,表示起飞，有一个竖直向上的合加速度，
      | 方向与NED系的D方向相反
  ch3 : Inport
  Add : Sum  Commented=on
  Constant2 : Constant  Commented=on  Value=0
  Constant4 : Constant  Value=0
  Gain : Gain  Commented=on  Gain=-1
  Memory1 : Memory
  Saturation1 : Saturate  UpperLimit=1  LowerLimit=0
  Scope1 : Scope  Commented=on
  Subsystem : Subsystem  Commented=on
  Subsystem1 : Subsystem
  Switch1 : Switch  Commented=on  Criteria=u2 > Threshold  SaturateOnIntegerOverflow=off  InputSameDT=off
  Switch2 : Switch  Criteria=u2 > Threshold  SaturateOnIntegerOverflow=off  InputSameDT=off
  g : Constant  Commented=on  Value=9.5
  weight : Outport
  wires:
  Constant2/1 -> Switch1/3
  Gain/1 -> Switch1/2
  Switch1/1 -> Subsystem/Trigger
  Switch2/1 -> weight/1
  Constant4/1 -> Switch2/3
  Saturation1/1 -> Switch2/1
  Memory1/1 -> Saturation1/1
  Subsystem/1(u) -> Scope1/1
  ch3/1 -> Memory1/1, Subsystem1/1(ch3)
  g/1 -> Add/2
  Add/1 -> Gain/1
  Subsystem1/1(u) -> Switch2/2

== system px4_controller_demo/Control System2/Phi Controler/PID2 ==
  Input : Inport
  weight : Inport  Port=2
  Add : Sum  Inputs=+++
  Discrete Derivative : simulink/Discrete/Discrete Derivative  gainval=1.0  ICPrevScaledInput=0.0  OutMin=[]  OutMax=[]  OutDataType=fixdt(1, 16)  OutScaling=2^-10  DoSatur=off
  Gain : Gain  Gain=0.8
  Gain1 : Gain  Gain=0.03
  积分限幅 : Subsystem
  Output : Outport
  wires:
  Gain1/1 -> Discrete Derivative/1
  Input/1 -> Gain1/1, Gain/1, 积分限幅/1(erro)
  积分限幅/1(Out1) -> Add/2
  Gain/1 -> Add/1
  Discrete Derivative/1 -> Add/3
  Add/1 -> Output/1
  weight/1 -> 积分限幅/2(weight)

== system px4_controller_demo/Control System2/Psi Controler/PI1 ==
  u : Inport
  weight : Inport  Port=2
  Add : Sum
  Display : Display
  Display1 : Display
  Gain1 : Gain  Commented=on  Gain=1.4  RndMeth=Nearest
  KP : Gain  Gain=1.4
  积分限幅 : Subsystem
  yaw_rate : Outport
  wires:
  积分限幅/1(I_out) -> Display1/1, Add/2
  weight/1 -> 积分限幅/2(erro)
  u/1 -> KP/1, 积分限幅/1(weight)
  KP/1 -> Display/1, Add/1
  Add/1 -> yaw_rate/1

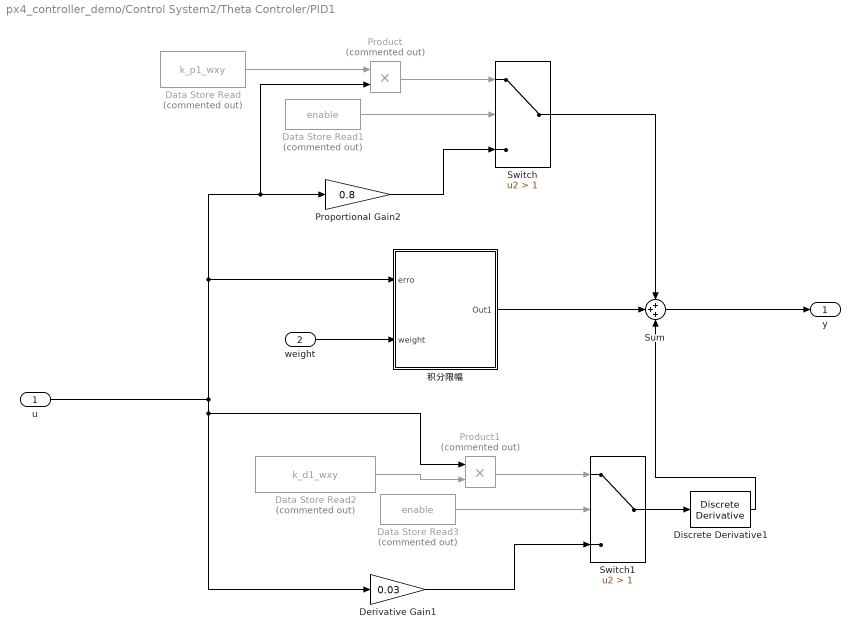
== system px4_controller_demo/Control System2/Theta Controler/PID1 ==
  u : Inport  SampleTime=dt
  "weight " : Inport  Port=2  SampleTime=dt
  Data Store Read : DataStoreRead  Commented=on  DataStoreName=k_p1_wxy  IndexOptions=Index vector (dialog)  Indices=1  OutputSizes=1
  Data Store Read1 : DataStoreRead  Commented=on  DataStoreName=enable  IndexOptions=Index vector (dialog)  Indices=1  OutputSizes=1
  Data Store Read2 : DataStoreRead  Commented=on  DataStoreName=k_d1_wxy  IndexOptions=Index vector (dialog)  Indices=1  OutputSizes=1
  Data Store Read3 : DataStoreRead  Commented=on  DataStoreName=enable  IndexOptions=Index vector (dialog)  Indices=1  OutputSizes=1
  Derivative Gain1 : Gain  DisableCoverage=on  Gain=0.03  SampleTime=dt
  Discrete Derivative1 : simulink/Discrete/Discrete Derivative  gainval=1.0  ICPrevScaledInput=0.0  OutMin=[]  OutMax=[]  OutDataType=fixdt(1, 16)  OutScaling=2^-10  DoSatur=off
  Product : Product  Commented=on
  Product1 : Product  Commented=on
  Proportional Gain2 : Gain  Gain=0.8  SampleTime=dt
  Sum : Sum  Inputs=+++  SampleTime=dt
  Switch : Switch  Criteria=u2 > Threshold  Threshold=1  SaturateOnIntegerOverflow=off  InputSameDT=off
  Switch1 : Switch  Criteria=u2 > Threshold  Threshold=1  SaturateOnIntegerOverflow=off  InputSameDT=off
  积分限幅 : Subsystem
  y : Outport  SampleTime=dt  InitialOutput=0
  wires:
  Data Store Read3/1 -> Switch1/2
  Derivative Gain1/1 -> Switch1/3
  Product1/1 -> Switch1/1
  u/1 -> 积分限幅/1(erro), Product/2, Proportional Gain2/1, Derivative Gain1/1, Product1/1
  Switch1/1 -> Discrete Derivative1/1
  Discrete Derivative1/1 -> Sum/3
  Data Store Read2/1 -> Product1/2
  积分限幅/1(Out1) -> Sum/2
  "weight "/1 -> 积分限幅/2("weight ")
  Proportional Gain2/1 -> Switch/3
  Switch/1 -> Sum/1
  Data Store Read1/1 -> Switch/2
  Product/1 -> Switch/1
  Data Store Read/1 -> Product/1
  Sum/1 -> y/1

== system px4_controller_demo/Control System2/Theta Controler/PID2 ==
  Input : Inport
  weight : Inport  Port=2
  Add : Sum  Inputs=+++
  Discrete Derivative : simulink/Discrete/Discrete Derivative  gainval=1.0  ICPrevScaledInput=0.0  OutMin=[]  OutMax=[]  OutDataType=fixdt(1, 16)  OutScaling=2^-10  DoSatur=off
  Gain : Gain  Gain=0.8
  Gain1 : Gain  Gain=0.03
  积分限幅 : Subsystem
  Output : Outport
  wires:
  Gain1/1 -> Discrete Derivative/1
  Input/1 -> Gain1/1, Gain/1, 积分限幅/1(erro)
  积分限幅/1(Out1) -> Add/2
  Gain/1 -> Add/1
  Discrete Derivative/1 -> Add/3
  Add/1 -> Output/1
  weight/1 -> 积分限幅/2(weight)

== system px4_controller_demo/Control System2/logical1/Subsystem ==
  In1 : Inport
  Trigger : TriggerPort  VariantControl=Variant  PortDimensions=1
  MATLAB Function : MATLAB Function  TreatAsAtomicUnit=on
  u : Outport
  wires:
  MATLAB Function/1(u) -> u/1
  In1/1 -> MATLAB Function/1(ch3)

== system px4_controller_demo/Control System2/logical1/Subsystem1 ==
  ch3 : Inport
  MATLAB Function : MATLAB Function  TreatAsAtomicUnit=on
  u : Outport
  wires:
  ch3/1 -> MATLAB Function/1(ch3)
  MATLAB Function/1(u) -> u/1

== system px4_controller_demo/Control System2/Phi Controler/PID2/积分限幅 ==
  erro : Inport
  weight : Inport  Port=2
  Compare To Constant : simulink/Logic and Bit Operations/Compare To Constant  relop=<=  const=0.05  OutDataTypeStr=boolean
  Integrator : DiscreteIntegrator  ExternalReset=level  SampleTime=-1  ICPrevOutput=DiscIntNeverNeededParam  ICPrevScaledInput=DiscIntNeverNeededParam
  Product3 : Product
  Proportional Gain1 : Gain  Gain=1.2
  i_factor1 : Subsystem
  satuation 1 : MATLAB Function  TreatAsAtomicUnit=on
  Out1 : Outport
  wires:
  Compare To Constant/1 -> Integrator/2
  Proportional Gain1/1 -> Integrator/1
  erro/1 -> i_factor1/1(In1), Product3/2
  satuation 1/1(y) -> Out1/1
  Integrator/1 -> satuation 1/1(u)  "ll"
  i_factor1/1(Out1) -> Product3/1
  Product3/1 -> Proportional Gain1/1
  weight/1 -> satuation 1/2(weight), Compare To Constant/1

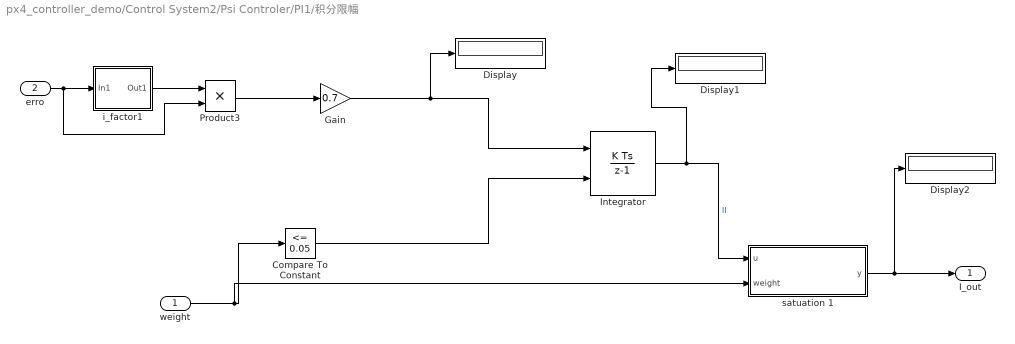
== system px4_controller_demo/Control System2/Psi Controler/PI1/积分限幅 ==
  weight : Inport
  erro : Inport  Port=2
  Compare To Constant : simulink/Logic and Bit Operations/Compare To Constant  relop=<=  const=0.05  OutDataTypeStr=boolean
  Display : Display
  Display1 : Display
  Display2 : Display
  Gain : Gain  Gain=0.7
  Integrator : DiscreteIntegrator  ExternalReset=level  SampleTime=-1  ICPrevOutput=DiscIntNeverNeededParam  ICPrevScaledInput=DiscIntNeverNeededParam
  Product3 : Product
  i_factor1 : Subsystem
  satuation 1 : MATLAB Function  TreatAsAtomicUnit=on
  I_out : Outport
  wires:
  erro/1 -> i_factor1/1(In1), Product3/2
  i_factor1/1(Out1) -> Product3/1
  Product3/1 -> Gain/1
  Gain/1 -> Display/1, Integrator/1
  Integrator/1 -> Display1/1, satuation 1/1(u)  "ll"
  satuation 1/1(y) -> Display2/1, I_out/1
  Compare To Constant/1 -> Integrator/2
  weight/1 -> satuation 1/2(weight), Compare To Constant/1

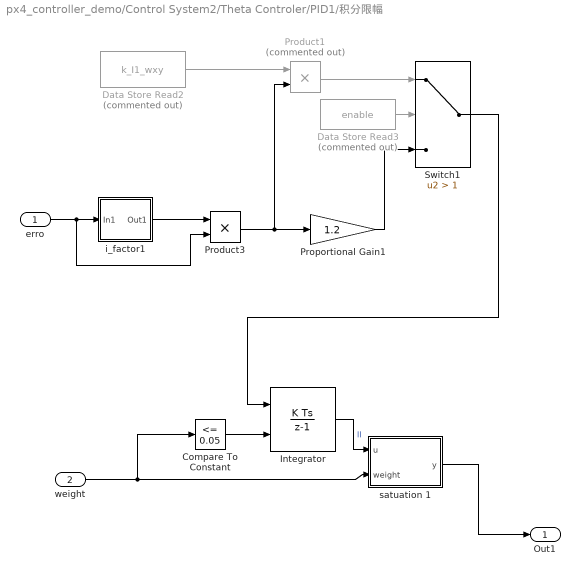
== system px4_controller_demo/Control System2/Theta Controler/PID1/积分限幅 ==
  erro : Inport
  "weight " : Inport  Port=2  SampleTime=dt
  Compare To Constant : simulink/Logic and Bit Operations/Compare To Constant  relop=<=  const=0.05  OutDataTypeStr=boolean
  Data Store Read2 : DataStoreRead  Commented=on  DataStoreName=k_I1_wxy  IndexOptions=Index vector (dialog)  Indices=1  OutputSizes=1
  Data Store Read3 : DataStoreRead  Commented=on  DataStoreName=enable  IndexOptions=Index vector (dialog)  Indices=1  OutputSizes=1
  Integrator : DiscreteIntegrator  ExternalReset=level  SampleTime=-1  ICPrevOutput=DiscIntNeverNeededParam  ICPrevScaledInput=DiscIntNeverNeededParam
  Product1 : Product  Commented=on
  Product3 : Product
  Proportional Gain1 : Gain  Gain=1.2  SampleTime=dt
  Switch1 : Switch  Criteria=u2 > Threshold  Threshold=1  SaturateOnIntegerOverflow=off  InputSameDT=off
  i_factor1 : Subsystem
  satuation 1 : MATLAB Function  TreatAsAtomicUnit=on
  Out1 : Outport
  wires:
  Compare To Constant/1 -> Integrator/2
  Switch1/1 -> Integrator/1
  erro/1 -> i_factor1/1(In1), Product3/2
  satuation 1/1(y) -> Out1/1
  Proportional Gain1/1 -> Switch1/3
  Integrator/1 -> satuation 1/1(u)  "ll"
  Product1/1 -> Switch1/1
  Data Store Read3/1 -> Switch1/2
  Data Store Read2/1 -> Product1/1
  "weight "/1 -> Compare To Constant/1, satuation 1/2(weight)
  i_factor1/1(Out1) -> Product3/1
  Product3/1 -> Proportional Gain1/1, Product1/2

== system px4_controller_demo/Control System2/Theta Controler/PID2/积分限幅 ==
  erro : Inport
  weight : Inport  Port=2
  Compare To Constant : simulink/Logic and Bit Operations/Compare To Constant  relop=<=  const=0.05  OutDataTypeStr=boolean
  Integrator : DiscreteIntegrator  ExternalReset=level  SampleTime=-1  ICPrevOutput=DiscIntNeverNeededParam  ICPrevScaledInput=DiscIntNeverNeededParam
  Product3 : Product
  Proportional Gain1 : Gain  Gain=1.2
  i_factor1 : Subsystem
  satuation 1 : MATLAB Function  TreatAsAtomicUnit=on
  Out1 : Outport
  wires:
  Compare To Constant/1 -> Integrator/2
  Proportional Gain1/1 -> Integrator/1
  erro/1 -> i_factor1/1(In1), Product3/2
  satuation 1/1(y) -> Out1/1
  Integrator/1 -> satuation 1/1(u)  "ll"
  i_factor1/1(Out1) -> Product3/1
  Product3/1 -> Proportional Gain1/1
  weight/1 -> satuation 1/2(weight), Compare To Constant/1

== system px4_controller_demo/Control System2/Phi Controler/PID2/积分限幅/i_factor1 ==
  In1 : Inport
  Add : Sum  Inputs=+-
  Constant : Constant  Value=150
  Constant1 : Constant
  Constant2 : Constant  Value=0
  Divide : Product  Inputs=*/
  Max : MinMax  Function=max  Inputs=2
  Product2 : Product
  Out1 : Outport
  wires:
  Constant1/1 -> Add/1
  Product2/1 -> Add/2
  In1/1 -> Divide/1
  Divide/1 -> Product2/2, Product2/1  "i_factor"
  Constant/1 -> Divide/2
  Max/1 -> Out1/1
  Constant2/1 -> Max/2
  Add/1 -> Max/1

== system px4_controller_demo/Control System2/Psi Controler/PI1/积分限幅/i_factor1 ==
  In1 : Inport
  Add : Sum  Inputs=+-
  Constant : Constant  Value=250
  Constant1 : Constant
  Constant2 : Constant  Value=0
  Divide : Product  Inputs=*/
  Max : MinMax  Function=max  Inputs=2
  Product2 : Product
  Out1 : Outport
  wires:
  Constant1/1 -> Add/1
  Product2/1 -> Add/2
  In1/1 -> Divide/1
  Divide/1 -> Product2/2, Product2/1  "i_factor"
  Constant/1 -> Divide/2
  Max/1 -> Out1/1
  Constant2/1 -> Max/2
  Add/1 -> Max/1

== system px4_controller_demo/Control System2/Theta Controler/PID1/积分限幅/i_factor1 ==
  In1 : Inport
  Add : Sum  Inputs=+-
  Constant : Constant  Value=150
  Constant1 : Constant
  Constant2 : Constant  Value=0
  Divide : Product  Inputs=*/
  Max : MinMax  Function=max  Inputs=2
  Product2 : Product
  Out1 : Outport
  wires:
  Constant1/1 -> Add/1
  Product2/1 -> Add/2
  In1/1 -> Divide/1
  Divide/1 -> Product2/2, Product2/1  "i_factor"
  Constant/1 -> Divide/2
  Max/1 -> Out1/1
  Constant2/1 -> Max/2
  Add/1 -> Max/1

== system px4_controller_demo/Control System2/Theta Controler/PID2/积分限幅/i_factor1 ==
  In1 : Inport
  Add : Sum  Inputs=+-
  Constant : Constant  Value=150
  Constant1 : Constant
  Constant2 : Constant  Value=0
  Divide : Product  Inputs=*/
  Max : MinMax  Function=max  Inputs=2
  Product2 : Product
  Out1 : Outport
  wires:
  Constant1/1 -> Add/1
  Product2/1 -> Add/2
  In1/1 -> Divide/1
  Divide/1 -> Product2/2, Product2/1  "i_factor"
  Constant/1 -> Divide/2
  Max/1 -> Out1/1
  Constant2/1 -> Max/2
  Add/1 -> Max/1

== matlab function px4_controller_demo/c_ch4_norm/MATLAB Function2 ==
  data: u input; y output
function y = fcn(u)
%[0,1]-->[-1,1]

y1 = u-0.5;
y = y1*2;
end

== matlab function px4_controller_demo/Control System2/Theta Controler/PID1/积分限幅/satuation 1 ==
  data: u input; y output; weight input
function y = fcn(u,weight)
if weight==0
    y=0;
else
    if u > 200*weight
        y = 200*weight;
    elseif u < -200*weight
        y = -200*weight;
    else
        y = u;
    end
end

== matlab function px4_controller_demo/c_ch2_norm/MATLAB Function2 ==
  data: u input; y output
function y = fcn(u)
%[0,1]-->[-1,1]

y1 = u-0.5;
y = y1*2;
end

== matlab function px4_controller_demo/Control System2/Phi Controler/PID2/积分限幅/satuation 1 ==
  data: u input; y output; weight input
function y = fcn(u,weight)
if weight==0
    y=0;
else
    if u > 200*weight
        y = 200*weight;
    elseif u < -200*weight
        y = -200*weight;
    else
        y = u;
    end
end

== matlab function px4_controller_demo/c_ch1_norm/MATLAB Function2 ==
  data: u input; y output
function y = fcn(u)
%[0,1]-->[-1,1]

y1 = u-0.5;
y = y1*2;
end

== matlab function px4_controller_demo/Control System2/Control_mix ==
  data: rol input; motor output; pit input; yaw input; thr input
function motor = sd(rol,pit,yaw,thr)
% 
% 	y1 =double( thr - rol + pit + yaw)*k;
% 	y2 =double( thr +rol +pit -yaw)*k;
% 	y3 =double( thr +rol -pit +yaw)*k;
% 	y4 =double( thr -rol -pit -yaw)*k;
%     motor = [y1;y2;y3;y4];
% 	y1 =double( thr - rol + pit + yaw);%后右下系下，1、3电机逆时针
% 	y2 =double( thr +rol +pit -yaw);
% 	y3 =double( thr +rol -pit +yaw);
% 	y4 =double( thr -rol -pit -yaw);
%     motor = [y1;y2;y3;y4];
y1 =double( thr +rol + pit + yaw);  %NED系下，1、3电机逆时针(按照机头指向，左上为1号，右上2号，右下3号，左下4号)
y2 =double( thr -rol +pit -yaw);
y3 =double( thr -rol -pit +yaw);
y4 =double( thr +rol -pit -yaw);
 motor = [y1;y2;y3;y4];

%--------------------------------------------------------------------------------------
% 二. 假如控制模块真是基于后（x）-右（y）-下(z)坐标系进行控制的，
%  那对应该混控算法的电机号及转序应为：
%             1       2
%               \    /---(右，东方)
%               /    \
%             4        3
% 4个电机转序为：从上往下看2、4号电机顺时针转动；1、3逆时针，自己推理的与CSDN一致

%总结：上述两种情况，z轴朝地时（右手一握，顺时针），
%从上往下看逆时针转动的俩电机产生正的控制yaw量（空气给旋翼的是顺时针扭矩)
%不管机体坐标系如何变换，确定偏航通道的控制量正负时一定先要先明确4个电机的转序！

== matlab function px4_controller_demo/Control System2/Theta Controler/PID2/积分限幅/satuation 1 ==
  data: u input; y output; weight input
function y = fcn(u,weight)
if weight<=0.05
    y=0;
else
    if u > 200*weight
        y = 200*weight;
    elseif u < -200*weight
        y = -200*weight;
    else
        y = u;
    end
end

== matlab function px4_controller_demo/Control System2/Psi Controler/PI1/积分限幅/satuation 1 ==
  data: u input; y output; weight input
function y = fcn(u,weight)
if weight==0
    y=0;
else
    if u > 200*weight
        y = 200*weight;
    elseif u < -200*weight
        y = -200*weight;
    else
        y = u;
    end
end

== matlab function px4_controller_demo/Control System2/Psi Controler/MATLAB Function2 ==
  data: x input; exp_yawrate output; ref input; zoom input
function exp_yawrate = fcn(x,ref,zoom)   %x==yawRateCmd
if(x>ref)   % 0<x<=1
    t = x - zoom;
    if(t<ref)
        t = ref;
    else
        t=x
    end
    
else   %    -1<=x<0
    t = x + zoom;
    if(t>ref)
        t = ref;
    else
        t=x;
    end
end
exp_yawrate = t*200;

== matlab function px4_controller_demo/Control System2/logical1/Subsystem/MATLAB Function ==
  data: ch3 input; u output
function u = fcn(ch3)
if(ch3>0.2)
    u=1;
else
    u=0;
end

== matlab function px4_controller_demo/Control System2/logical1/Subsystem1/MATLAB Function ==
  data: ch3 input; u output
function u = fcn(ch3)
if(ch3>0.3)
    u=1;
else
    u=0;
end
